simulink model "MultiRobotSim"  (R2021b)
settings: Solver=FixedStepAuto  StartTime=0.0  StopTime=inf  FixedStep=sampleTime  RelTol=1e-3
PreLoadFcn:
  | % Simulation parameters
  | load exampleMap
  | sampleTime = 0.05;
  | 
  | % Robot parameters
  | wheelRadius = 0.025;
  | robotRadius = 0.35;
  | 
  | % Lidar parameters
  | sensorOffset = [0,0];
  | scanAngles = linspace(-pi/2,pi/2,9)';
  | maxRange = 5;
libraries: mobileRoboticsLib x13
settings Model: SimulationMode=accelerator  Creator=scastro  LastModifiedBy=vamse
settings SolverCC: AlgebraicLoopSolver=TrustRegion
settings DataIOCC: ReturnWorkspaceOutputs=off
settings DebuggingCC: PregeneratedLibrarySubsystemCodeDiagnostic=none  SFMachineParentedDataDiag=warning  ArithmeticOperatorsInVariantConditions=warning
settings SFSimCC: SimUseLocalCustomCode=off  CustomCodeUndefinedFunction=UseInterfaceOnly
settings RTWCC: RTWUseLocalCustomCode=off

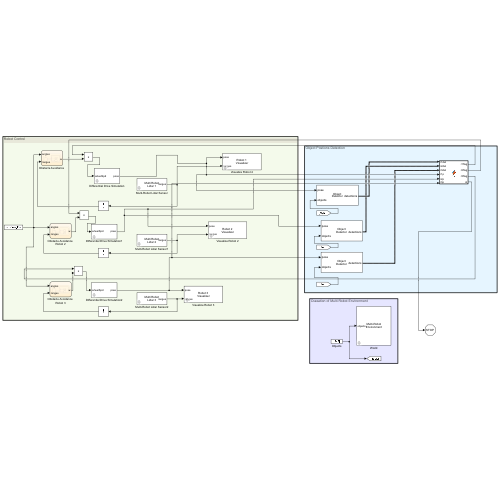
[thumbnail: Simulink's stored preview of the top-level diagram]
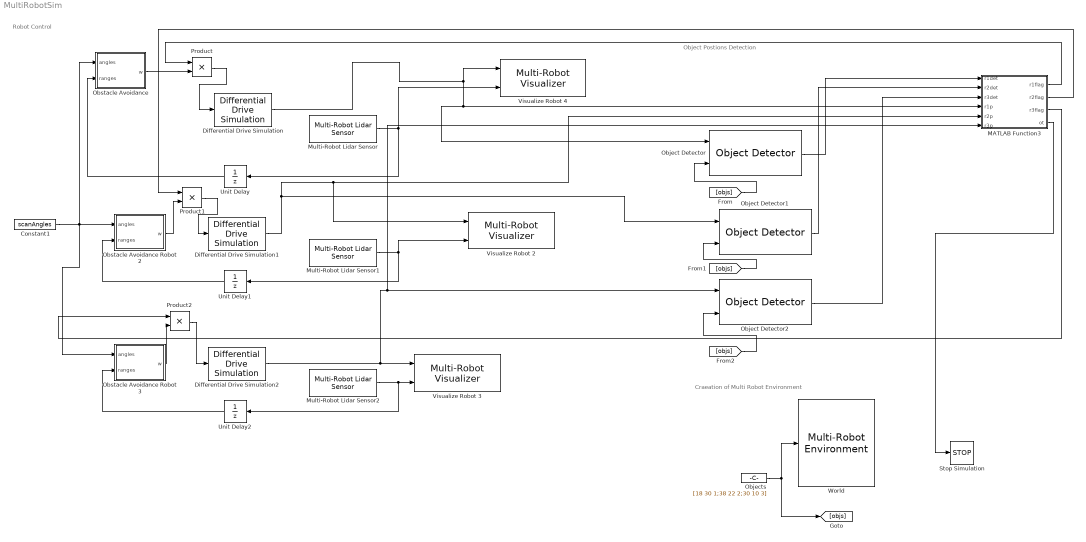
== system MultiRobotSim ==
  note: Robot Control
  note: Object Postions Detection
  note: Craeation of Multi Robot Environment
  Constant1 : Constant  Value=scanAngles
  Differential Drive Simulation : mobileRoboticsLib/Kinematic Models/Differential Drive/Differential Drive Simulation  wheelRadius=wheelRadius  wheelBase=robotRadius  initX=47  initY=3  initAngle=0  Ts=sampleTime
      settings: SourceProductName=Mobile Robotics Simulation Toolbox
  Differential Drive Simulation1 : mobileRoboticsLib/Kinematic Models/Differential Drive/Differential Drive Simulation  wheelRadius=wheelRadius  wheelBase=robotRadius  initX=5  initY=37  initAngle=0  Ts=sampleTime
      settings: SourceProductName=Mobile Robotics Simulation Toolbox
  Differential Drive Simulation2 : mobileRoboticsLib/Kinematic Models/Differential Drive/Differential Drive Simulation  wheelRadius=wheelRadius  wheelBase=robotRadius  initX=48  initY=39  initAngle=0  Ts=sampleTime
      settings: SourceProductName=Mobile Robotics Simulation Toolbox
  MATLAB Function3 : MATLAB Function  TreatAsAtomicUnit=on
  Multi-Robot Lidar Sensor : mobileRoboticsLib/Environments/Multi-Robot Lidar Sensor  robotIdx=1  mapName=map  sensorOffset=sensorOffset  scanAngles=scanAngles  maxRange=maxRange
      settings: SourceProductName=Mobile Robotics Simulation Toolbox
  Multi-Robot Lidar Sensor1 : mobileRoboticsLib/Environments/Multi-Robot Lidar Sensor  robotIdx=2  mapName=map  sensorOffset=sensorOffset  scanAngles=scanAngles  maxRange=maxRange
      settings: SourceProductName=Mobile Robotics Simulation Toolbox
  Multi-Robot Lidar Sensor2 : mobileRoboticsLib/Environments/Multi-Robot Lidar Sensor  robotIdx=3  mapName=map  sensorOffset=sensorOffset  scanAngles=scanAngles  maxRange=maxRange
      settings: SourceProductName=Mobile Robotics Simulation Toolbox
  Object Detector : mobileRoboticsLib/Environments/Object Detector  sensorOffset=[ 0, 0 ]  sensorAngle=0  fieldOfView=pi/3  maxRange=4  maxDetections=5  sampleTime=0.1
      settings: SourceProductName=Mobile Robotics Simulation Toolbox
  Object Detector1 : mobileRoboticsLib/Environments/Object Detector  sensorOffset=[ 0, 0 ]  sensorAngle=0  fieldOfView=pi/3  maxRange=4  maxDetections=5  sampleTime=0.1
      settings: SourceProductName=Mobile Robotics Simulation Toolbox
  Object Detector2 : mobileRoboticsLib/Environments/Object Detector  sensorOffset=[ 0, 0 ]  sensorAngle=0  fieldOfView=pi/3  maxRange=4  maxDetections=5  sampleTime=0.1
      settings: SourceProductName=Mobile Robotics Simulation Toolbox
  Objects : Constant  Value=[18 30 1;38 22 2;30 10 3]
  "Obstacle Avoidance " : Stateflow chart  TreatAsAtomicUnit=on
  Obstacle Avoidance Robot 2 : Stateflow chart  TreatAsAtomicUnit=on
  Obstacle Avoidance Robot 3 : Stateflow chart  TreatAsAtomicUnit=on
  Product : Product
  Product1 : Product
  Product2 : Product
  Stop Simulation : Stop
  Unit Delay : UnitDelay  SampleTime=-1  HasFrameUpgradeWarning=on
  Unit Delay1 : UnitDelay  SampleTime=-1  HasFrameUpgradeWarning=on
  Unit Delay2 : UnitDelay  SampleTime=-1  HasFrameUpgradeWarning=on
  Visualize Robot 2 : mobileRoboticsLib/Environments/Multi-Robot Visualizer  idx=2  radius=robotRadius  robotColor=[0 0 1]  showTraj=on  hasLidar=on  sensorOffset=sensorOffset  scanAngles=scanAngles  maxNumScans=0  hasObjDetector=on  objDetectorOffset=objDetectorOffset  objDetectorAngle=objDetectorAngle  objDetectorFOV=objDetectorFOV  objDetectorMaxRange=objDetectorRange  hasRobotDetector=off  robotDetectorOffset=[0,0]  robotDetectorAngle=0  robotDetectorFOV=pi/3  robotDetectorMaxRange=5  robotDetectorNumDetections=0
      settings: SourceProductName=Mobile Robotics Simulation Toolbox
  Visualize Robot 3 : mobileRoboticsLib/Environments/Multi-Robot Visualizer  idx=3  radius=robotRadius  robotColor=[0 0 1]  showTraj=on  hasLidar=on  sensorOffset=sensorOffset  scanAngles=scanAngles  maxNumScans=0  hasObjDetector=on  objDetectorOffset=objDetectorOffset  objDetectorAngle=objDetectorAngle  objDetectorFOV=objDetectorFOV  objDetectorMaxRange=objDetectorRange  hasRobotDetector=off  robotDetectorOffset=[0,0]  robotDetectorAngle=0  robotDetectorFOV=pi/3  robotDetectorMaxRange=5  robotDetectorNumDetections=0
      settings: SourceProductName=Mobile Robotics Simulation Toolbox
  Visualize Robot 4 : mobileRoboticsLib/Environments/Multi-Robot Visualizer  idx=1  radius=0  robotColor=[0 0 1]  showTraj=on  hasLidar=on  sensorOffset=sensorOffset  scanAngles=scanAngles  maxNumScans=0  hasObjDetector=on  objDetectorOffset=objDetectorOffset  objDetectorAngle=objDetectorAngle  objDetectorFOV=objDetectorFOV  objDetectorMaxRange=objDetectorRange  hasRobotDetector=off  robotDetectorOffset=[0,0]  robotDetectorAngle=0  robotDetectorFOV=pi/3  robotDetectorMaxRange=5  robotDetectorNumDetections=0
      settings: SourceProductName=Mobile Robotics Simulation Toolbox
  World : mobileRoboticsLib/Environments/Multi-Robot Environment  numRobots=3  mapName=map  showWaypoints=off  showObjects=on  objectColors=[1 0 0;0 1 0;0 0 1]  objectMarkers='so^'  showRobotIds=on  plotSensorLines=on
      settings: SourceProductName=Mobile Robotics Simulation Toolbox
  wires:
  "Obstacle Avoidance "/1(w) -> Product/2
  Unit Delay/1 -> "Obstacle Avoidance "/2(ranges)
  Unit Delay1/1 -> Obstacle Avoidance Robot 2/2(ranges)
  Unit Delay2/1 -> Obstacle Avoidance Robot 3/2(ranges)
  Constant1/1 -> Obstacle Avoidance Robot 3/1(angles), Obstacle Avoidance Robot 2/1(angles), "Obstacle Avoidance "/1(angles)
  Multi-Robot Lidar Sensor2/1 -> Visualize Robot 3/2, Unit Delay2/1
  Multi-Robot Lidar Sensor/1 -> Visualize Robot 4/2, Unit Delay/1
  Multi-Robot Lidar Sensor1/1 -> Unit Delay1/1, Visualize Robot 2/2
  Objects/1 -> World/1, [objs]
  [objs] -> Object Detector/2
  Object Detector/1 -> MATLAB Function3/1(r1det)
  [objs] -> Object Detector1/2
  [objs] -> Object Detector2/2
  Differential Drive Simulation2/1 -> Visualize Robot 3/1, MATLAB Function3/6(r3p), Object Detector2/1
  Product/1 -> Differential Drive Simulation/1
  Product1/1 -> Differential Drive Simulation1/1
  Object Detector1/1 -> MATLAB Function3/2(r2det)
  Obstacle Avoidance Robot 2/1(w) -> Product1/2
  Product2/1 -> Differential Drive Simulation2/1
  Object Detector2/1 -> MATLAB Function3/3(r3det)
  Obstacle Avoidance Robot 3/1(w) -> Product2/2
  MATLAB Function3/1(r1flag) -> Product/1
  MATLAB Function3/2(r2flag) -> Product1/1
  MATLAB Function3/3(r3flag) -> Product2/1
  Differential Drive Simulation1/1 -> MATLAB Function3/5(r2p), Visualize Robot 2/1, Object Detector1/1
  Differential Drive Simulation/1 -> Object Detector/1, MATLAB Function3/4(r1p), Visualize Robot 4/1
  MATLAB Function3/4(ot) -> Stop Simulation/1

== matlab function MultiRobotSim/MATLAB Function3 ==
  data: r1det input; r1flag output; r2det input; r3det input; r2flag output; r3flag output; r1p input; r2p input; r3p input; ot output
function [r1flag,r2flag,r3flag,ot]= fcn(r1det,r2det,r3det,r1p,r2p,r3p)
persistent poseMat
persistent count

if isempty(poseMat)
  poseMat = zeros(3,3);
end
count=0;
ot=0;
r1flag=1;
r2flag=1;
r3flag=1;

if ~isempty(r1det)
   r1flag=0;
   
   count=count+1
   i=r1det(3)
   poseMat(i,1)=r1p(1)
   poseMat(i,2)=r1p(2)
   poseMat(i,3)=r1p(3)
end   
if ~isempty(r2det)
   r2flag=0;
   count=count+1
   i=r2det(3);
   poseMat(i,1)=r2p(1)
   poseMat(i,2)=r2p(2)
   poseMat(i,3)=r2p(3)
end 
if ~isempty(r3det)
   r3flag=0;
   count=count+1
    i=r3det(3)
   poseMat(i,1)=r3p(1)
   poseMat(i,2)=r3p(2)
   poseMat(i,3)=r3p(3)
end
if (count==3)
    ot=1
end

== stateflow chart MultiRobotSim/Obstacle Avoidance Robot 2 ==
  state MainState [parallel]
    en,du:
    validIdx = ~isnan(ranges);
    validRanges = ranges(validIdx);
    validAngles = angles(validIdx);
    settings: executionOrder=1
    state Turn
      en,du:
      avgAngle = mean(validAngles./validRanges);
      state Left
        en, du:
        w = [0; 50.5];
      state Right
        en, du:
        w = [50.5;0];
      (default) -> (junction 39)
      (junction 39) -> Left [order 1] : [avgAngle < 0]
      (junction 39) -> (junction 43) [order 2]
      Left -> Right : [after(1,sec) && ...
          | avgAngle > 0]
      Right -> Left : [after(1,sec) && ...
          | avgAngle < 0]
      (junction 43) -> Right
    state GoStraight
      en:
      w = [300; 300];
    (default) -> GoStraight
    GoStraight -> Turn : [any(validRanges<=1)]
    Turn -> GoStraight : [all(validRanges>1)]
  data: angles input; w output; ranges input; validRanges local size=numel(scanAngles); validIdx local; validAngles local size=numel(scanAngles); avgAngle local

== stateflow chart MultiRobotSim/Obstacle Avoidance Robot 3 ==
  state MainState [parallel]
    en,du:
    validIdx = ~isnan(ranges);
    validRanges = ranges(validIdx);
    validAngles = angles(validIdx);
    settings: executionOrder=1
    state Turn
      en,du:
      avgAngle = mean(validAngles./validRanges);
      state Left
        en, du:
        w = [0;50.5];
      state Right
        en, du:
        w = [50.5;0];
      (default) -> (junction 39)
      (junction 39) -> Left [order 1] : [avgAngle < 0]
      (junction 39) -> (junction 43) [order 2]
      Left -> Right : [after(1,sec) && ...
          | avgAngle > 0]
      Right -> Left : [after(1,sec) && ...
          | avgAngle < 0]
      (junction 43) -> Right
    state GoStraight
      en:
      w = [300; 300];
    (default) -> GoStraight
    GoStraight -> Turn : [any(validRanges<=1)]
    Turn -> GoStraight : [all(validRanges>1)]
  data: angles input; w output; ranges input; validRanges local size=numel(scanAngles); validIdx local; validAngles local size=numel(scanAngles); avgAngle local

== stateflow chart MultiRobotSim/Obstacle Avoidance  ==
  state MainState [parallel]
    en,du:
    validIdx = ~isnan(ranges);
    validRanges = ranges(validIdx);
    validAngles = angles(validIdx);
    settings: executionOrder=1
    state Turn
      en,du:
      avgAngle = mean(validAngles./validRanges);
      state Left
        en, du:
        w = [0;50.5];
      state Right
        en, du:
        w = [50.5;0];
      (default) -> (junction 39)
      (junction 39) -> Left [order 1] : [avgAngle < 0]
      (junction 39) -> (junction 43) [order 2]
      Left -> Right : [after(1,sec) && ...
          | avgAngle > 0]
      Right -> Left : [after(1,sec) && ...
          | avgAngle < 0]
      (junction 43) -> Right
    state GoStraight
      en:
      w = [250; 250];
    (default) -> GoStraight
    GoStraight -> Turn : [any(validRanges<=1)]
    Turn -> GoStraight : [all(validRanges>1)]
  data: angles input; w output; ranges input; validRanges local size=numel(scanAngles); validIdx local; validAngles local size=numel(scanAngles); avgAngle local
